simulink model "tank_test"  (R2026a)
settings: Solver=ode15s
libraries: scuba_lib x3, nesl_utility x2, fl_lib x2
settings Model: Creator=grouleau  LastModifiedBy=grouleau

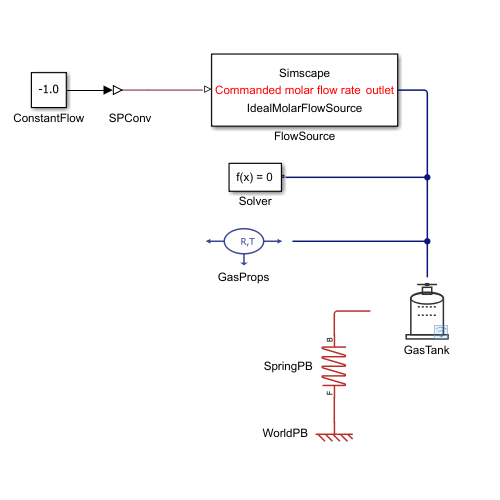
[thumbnail: Simulink's stored preview of the top-level diagram]
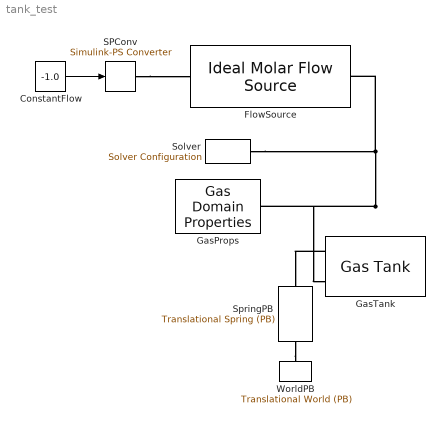
== system tank_test ==
  ConstantFlow : Constant  Value=-1.0
  FlowSource : scuba_lib/gas/elements/Ideal Molar Flow Source  n_dot_in_specify=off  n_dot_in_priority=None  n_dot_in=0 mol/s  n_dot_in_nominal_specify=off  n_dot_in_nominal_value=1  n_dot_in_nominal_unit=mol/s
  GasProps : scuba_lib/gas/elements/Gas Domain Properties  R_gas=8.314 J/(K*mol)  T=293.15 K  n_dot_thru_specify=off  n_dot_thru_priority=None  n_dot_thru=0 mol/s  n_dot_thru_nominal_specify=off  n_dot_thru_nominal_value=1  n_dot_thru_nominal_unit=mol/s
  GasTank : scuba_lib/gas/elements/Gas Tank  V_tank=0.012 m^3  n_init=98.47 mol  M_gas=0.029 kg/mol  n_dot_out_specify=off  n_dot_out_priority=None  n_dot_out=0 mol/s  n_dot_out_nominal_specify=off  n_dot_out_nominal_value=1  n_dot_out_nominal_unit=mol/s  f_specify=off  f_priority=None  f=0 N  f_nominal_specify=off  f_nominal_value=1  f_nominal_unit=N
  SPConv : nesl_utility/Simulink-PS Converter  PhysicalDomain=network_engine_domain  SubClassName=ps_input  LeftPortType=input  RightPortType=output  PseudoPeriodic=off  Frequencies=[]  NoiseDistribution=none  NoiseParameters=[]  Unit=1  AffineConversion=off  FilteringAndDerivatives=provide  SimscapeFilterOrder=1  InputFilterTimeConstant=0.001  UdotUserProvided=0
  Solver : nesl_utility/Solver Configuration  PhysicalDomain=network_engine_domain  SubClassName=solver  LeftPortType=input  RightPortType=generic  Tones=[]  Harmonics=[]  SimulateNoise=off  Profile=off  UseLocalSampling=off  EnableSwitchedLinearOptims=on  FrequencyDomain=off  UseCCode=off  RelTol=0.001  AbsTol=0.001  MinStep=1e-09  ToWorkspace=off  RevertToSquareIcSolve=off  NumHomotopyIterations=100  PhasorMode=off  PhasorModeNumHarmonics=1  ConsistencySolver=NEWTON_XTOL_AFTER_FTOL  CanonicalOrdering=CANONICAL  OptimizeIntermediates=OPTIMIZED  IndexReductionMethod=DerivativeReplacement  DoDC=off  ResidualTolerance=1e-09  ConsistencyTolSource=GLOBAL  ConsistencyAbsTol=0.001  ConsistencyRelTol=0.001  ConsistencyTolFactor=0.001  UseLocalSolver=off  LocalSolverChoice=NE_BACKWARD_EULER_ADVANCER  ResolveIndetEquations=on  FunctionEvalNumThread=1  LocalSolverSampleTime=0.001  DoFixedCost=off  MaxNonlinIter=3  MaxModeIter=2  ComputeImpulses=off  ImpulseIterations=2  LinearAlgebra=auto  LinearAlgebraNumThread=0  EquationFormulation=NE_TIME_EF  DelaysMemoryBudget=1024  AutomaticFiltering=on  FilteringTimeConstant=0.001  PartitionStorageMethod=AS_NEEDED  PartitionMemoryBudget=1024  PartitionMethod=ROBUST  MultibodyUseLocalSolver=off  MultibodyLocalSolverChoice=ODE1  MultibodyLocalSolverSampleTime=0.001
  SpringPB : fl_lib/Translational/Elements/Translational Spring (PB)  stiffness=1e3 N/m  f_specify=off  f_priority=None  f=0 N  f_nominal_specify=off  f_nominal_value=1  f_nominal_unit=N  deformation_specify=off  deformation_priority=None  deformation=0 m  deformation_nominal_specify=off  deformation_nominal_value=1  deformation_nominal_unit=m  length_specify=off  length_priority=None  length=0.1 m  length_nominal_specify=off  length_nominal_value=1  length_nominal_unit=m  rest_length_specify=off  rest_length_priority=None  rest_length=0.1 m  rest_length_nominal_specify=off  rest_length_nominal_value=1  rest_length_nominal_unit=m
  WorldPB : fl_lib/Translational/Elements/Translational World (PB)
  wires:
  ConstantFlow/1 -> SPConv/1
  connections:
  GasTank/LConn1 -- SpringPB/LConn1
  SpringPB/RConn1 -- WorldPB/RConn1
  SPConv/RConn1 -- FlowSource/LConn1
  Solver/RConn1 -- GasProps/LConn1 -- GasTank/LConn2 -- FlowSource/RConn1
